simulink model "accs_ut"  (Simulink 8.1)
settings: Solver=FixedStepDiscrete  StartTime=0.0  StopTime=Inf  FixedStep=0.005  RelTol=1e-3
libraries: siltestlib x18, accs x1
settings Model: Creator=AT015555  LastModifiedBy=AT015555
settings DataIOCC: SignalLoggingSaveFormat=Dataset
settings OptimizationCC: ExpressionDepthLimit=128
settings DebuggingCC: FcnCallInpInsideContextMsg=EnableAllAsError
settings GRTTargetCC: CombineOutputUpdateFcns=on  GRTInterface=off

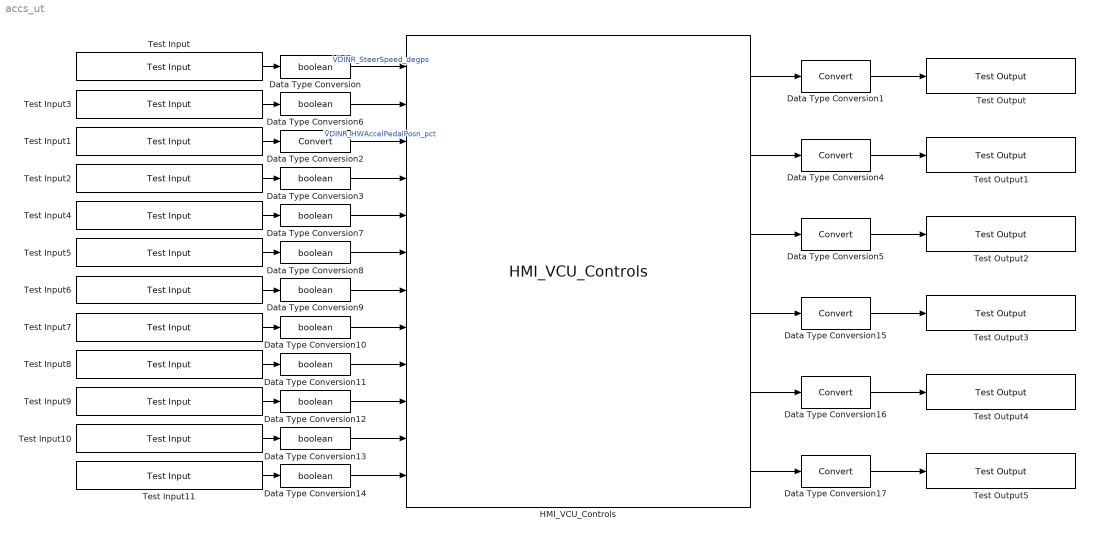
== system accs_ut ==
  Data Type Conversion{,3,6..14} (11 alike) : DataTypeConversion  OutDataTypeStr=boolean
  Data Type Conversion{1..2,4..5,15..17} (7 alike) : DataTypeConversion
  HMI_VCU_Controls : accs/HMI_VCU_Controls
  Test Input : siltestlib/Test Input  varname=VDINR_ACCOnVCU_flg  sampletime=0.005
  Test Input1 : siltestlib/Test Input  varname=VACC_ACCSystemStatePrev_enum  sampletime=0.005
  Test Input10 : siltestlib/Test Input  varname=VDINR_ACCDistVCU_flg  sampletime=0.005
  Test Input11 : siltestlib/Test Input  varname=VDINR_ACCTimeGapDecH_flg  sampletime=0.005
  Test Input2 : siltestlib/Test Input  varname=VACC_ACCActingPrev_flg  sampletime=0.005
  Test Input3 : siltestlib/Test Input  varname=VDINR_ACCOnH_flg  sampletime=0.005
  Test Input4 : siltestlib/Test Input  varname=VDINR_ACCSetSpdDecH_flg  sampletime=0.005
  Test Input5 : siltestlib/Test Input  varname=VDINR_ACCSpdDecH_flg  sampletime=0.005
  Test Input6 : siltestlib/Test Input  varname=VDINR_ACCResSpdIncH_flg  sampletime=0.005
  Test Input7 : siltestlib/Test Input  varname=VDINR_ACCSpdIncH_flg  sampletime=0.005
  Test Input8 : siltestlib/Test Input  varname=VDINR_ACCResSpdIncVCU_flg  sampletime=0.005
  Test Input9 : siltestlib/Test Input  varname=VDINR_ACCSpdDecVCU_flg  sampletime=0.005
  Test Output : siltestlib/Test Output  varname=VIFO_ACCTurnOnReq_flg  sampletime=-1
  Test Output1 : siltestlib/Test Output  varname=VIFO_ACCTurnOffReq_flg  sampletime=-1
  Test Output2 : siltestlib/Test Output  varname=VIFO_ACCCancelReq_flg  sampletime=-1
  Test Output3 : siltestlib/Test Output  varname=VIFO_ACCSetSpdDec_flg  sampletime=-1
  Test Output4 : siltestlib/Test Output  varname=VIFO_ACCResSpdInc_flg  sampletime=-1
  Test Output5 : siltestlib/Test Output  varname=VIFO_ACCDist_flg  sampletime=-1
  wires:
  Test Input/1 -> Data Type Conversion/1
  Test Input1/1 -> Data Type Conversion2/1
  Data Type Conversion1/1 -> Test Output/1
  HMI_VCU_Controls/1 -> Data Type Conversion1/1
  Test Input2/1 -> Data Type Conversion3/1
  Data Type Conversion4/1 -> Test Output1/1
  HMI_VCU_Controls/2 -> Data Type Conversion4/1
  Data Type Conversion5/1 -> Test Output2/1
  HMI_VCU_Controls/3 -> Data Type Conversion5/1
  Test Input3/1 -> Data Type Conversion6/1
  Data Type Conversion6/1 -> HMI_VCU_Controls/2
  Data Type Conversion3/1 -> HMI_VCU_Controls/4
  Data Type Conversion/1 -> HMI_VCU_Controls/1  "VDINR_SteerSpeed_degps"
  Data Type Conversion2/1 -> HMI_VCU_Controls/3  "VDINR_HWAccelPedalPosn_pct"
  Test Input4/1 -> Data Type Conversion7/1
  Test Input5/1 -> Data Type Conversion8/1
  Test Input6/1 -> Data Type Conversion9/1
  Test Input7/1 -> Data Type Conversion10/1
  Test Input8/1 -> Data Type Conversion11/1
  Test Input9/1 -> Data Type Conversion12/1
  Test Input10/1 -> Data Type Conversion13/1
  Test Input11/1 -> Data Type Conversion14/1
  Data Type Conversion9/1 -> HMI_VCU_Controls/7
  Data Type Conversion12/1 -> HMI_VCU_Controls/10
  Data Type Conversion8/1 -> HMI_VCU_Controls/6
  Data Type Conversion14/1 -> HMI_VCU_Controls/12
  Data Type Conversion10/1 -> HMI_VCU_Controls/8
  Data Type Conversion7/1 -> HMI_VCU_Controls/5
  Data Type Conversion11/1 -> HMI_VCU_Controls/9
  Data Type Conversion13/1 -> HMI_VCU_Controls/11
  Data Type Conversion15/1 -> Test Output3/1
  HMI_VCU_Controls/4 -> Data Type Conversion15/1
  Data Type Conversion16/1 -> Test Output4/1
  Data Type Conversion17/1 -> Test Output5/1
  HMI_VCU_Controls/5 -> Data Type Conversion16/1
  HMI_VCU_Controls/6 -> Data Type Conversion17/1
